simulink model "ARMAX_Obtencion_Datos_Primer_Orden_Con_Ruido"  (R2016a)
settings: Solver=VariableStepAuto  StartTime=0.0  StopTime=10.0  RelTol=1e-3
libraries: simulink x1
settings Model: Creator=Daniel  LastModifiedBy=Daniel

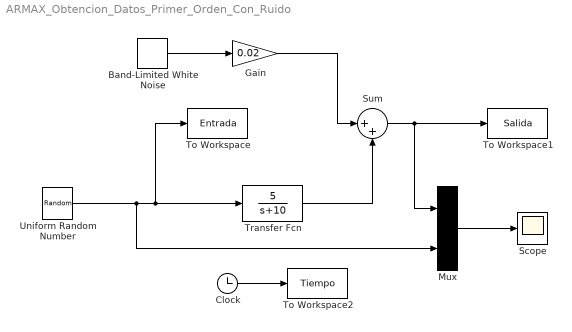
== system ARMAX_Obtencion_Datos_Primer_Orden_Con_Ruido ==
  Band-Limited White Noise : simulink/Sources/Band-Limited White Noise  Cov=[0.1]  Ts=0.01  seed=[23341]
  Clock : Clock
  Gain : Gain  Gain=0.02
  Mux : Mux  Inputs=2
  Scope : Scope
  Sum : Sum  Inputs=|++
  To Workspace : ToWorkspace  VariableName=Entrada  SampleTime=0.01
  To Workspace1 : ToWorkspace  VariableName=Salida  SampleTime=0.01
  To Workspace2 : ToWorkspace  VariableName=Tiempo  SampleTime=0.01
  Transfer Fcn : TransferFcn  Numerator=[5]  Denominator=[1 10]
  Uniform Random Number : UniformRandomNumber  Minimum=0  Maximum=5  SampleTime=0.5
  wires:
  Uniform Random Number/1 -> Mux/2, To Workspace/1, Transfer Fcn/1
  Transfer Fcn/1 -> Sum/2
  Mux/1 -> Scope/1
  Band-Limited White Noise/1 -> Gain/1
  Clock/1 -> To Workspace2/1
  Gain/1 -> Sum/1
  Sum/1 -> To Workspace1/1, Mux/1
